simulink model "controllerSim"  (R2018b)
settings: Solver=VariableStepAuto  StartTime=0.0  StopTime=10.0  RelTol=1e-3
PreLoadFcn:
  | initParams;
values from neighbouring files (symbols this model uses):
  b = 3.508E-5    (= 3.508e-05)    [initParams.m]
  J = 3.228E-6    (= 3.228e-06)    [initParams.m]
  K = 2.740E-4    (= 0.000274)    [initParams.m]
  L = 2.750E-5    (= 2.75e-05)    [initParams.m]
  R = 4    [initParams.m]
undefined symbols (not defined in the file or in its folder): sigbuilder_block
libraries: simulink_extras x1
settings Model: Creator=cdsouza  LastModifiedBy=cdsouza
settings DebuggingCC: LibraryContextMissingDiagnostic=none
settings SFSimCC: SimUseLocalCustomCode=off
settings RTWCC: RTWUseLocalCustomCode=off

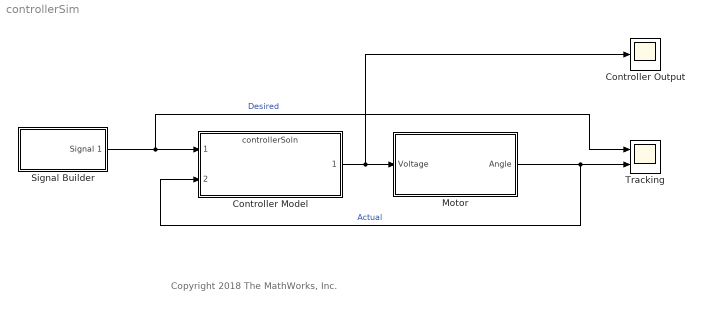
== system controllerSim ==
  note: Copyright 2018 The MathWorks, Inc.
  Controller Model : ModelReference  ModelNameDialog=controllerSoln  SimulationMode=Normal  ModelReferenceVersion=1.11
  Controller Output : Scope
  Motor : Subsystem  TreatAsAtomicUnit=on
  Signal Builder : Subsystem  Tag=STV Subsys  LoadFcn=sigbuilder_block('load');  StartFcn=sigbuilder_block('start');  StopFcn=sigbuilder_block('stop');  ClipboardFcn=sigbuilder_block('clipboard');  mask(Sigbuilder block){tuvar=[0:10]}
      mask help: Simulink:masks:SigbuilderBlock_MD
      mask init:
      | if ~strcmp(get_param(bdroot(gcbh),'SimulationStatus'),'stopped') tuvar = sigbuilder_block('maskInit'); end
      settings: CopyFcn=sigbuilder_block('copy');  DeleteFcn=sigbuilder_block('delete');  ModelCloseFcn=sigbuilder_block('modelClose');  PreSaveFcn=sigbuilder_block('preSave');  PauseFcn=sigbuilder_block('pause');  ContinueFcn=sigbuilder_block('continue');  NameChangeFcn=sigbuilder_block('namechange');  OpenFcn=sigbuilder_block('open',[436.966 199.241 549.931 400.345 ]);  CloseFcn=sigbuilder_block('close');
      mask Display: plot(0, 0, 100, 100,[2, 2, 32, 32, 2], [68, 8, 8, 68, 68],[32, 2], [38, 38], [32, 19, 2],[53, 60, 44], [32, 17, 17, 2],[16, 16, 31, 31]);txt = getActiveGroup(gcbh);text(2, 100, txt,'verticalAlignment', 'top');
  Tracking : Scope  NumInputPorts=2
  wires:
  Signal Builder/1(Signal 1) -> Tracking/1, Controller Model/1  "Desired"
  Motor/1(Angle) -> Controller Model/2, Tracking/2  "Actual"
  Controller Model/1 -> Controller Output/1, Motor/1(Voltage)

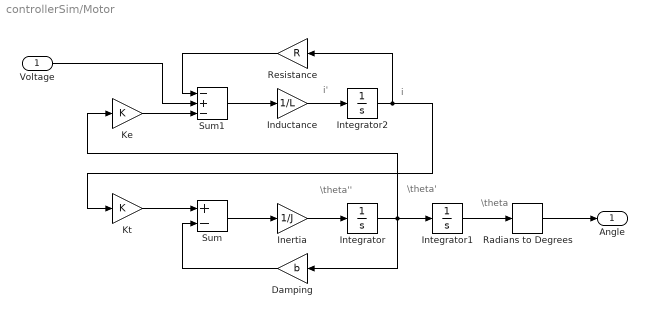
== system controllerSim/Motor ==
  note: \theta
  note: \theta''
  note: \theta'
  note: i
  note: i'
  Voltage : Inport
  Damping : Gain  Gain=b  SaturateOnIntegerOverflow=on  OutDataTypeStr=Inherit: Same as input  ParamDataTypeStr=Inherit: Same as input
  Inductance : Gain  Gain=1/L  SaturateOnIntegerOverflow=on  OutDataTypeStr=Inherit: Same as input  ParamDataTypeStr=Inherit: Same as input
  Inertia : Gain  Gain=1/J  SaturateOnIntegerOverflow=on  OutDataTypeStr=Inherit: Same as input  ParamDataTypeStr=Inherit: Same as input
  Integrator : Integrator
  Integrator1 : Integrator
  Integrator2 : Integrator
  Ke : Gain  Gain=K  SaturateOnIntegerOverflow=on  OutDataTypeStr=Inherit: Same as input  ParamDataTypeStr=Inherit: Same as input
  Kt : Gain  Gain=K  SaturateOnIntegerOverflow=on  OutDataTypeStr=Inherit: Same as input  ParamDataTypeStr=Inherit: Same as input
  Radians to Degrees : simulink_extras/Transformations/Radians to Degrees
  Resistance : Gain  Gain=R  SaturateOnIntegerOverflow=on  OutDataTypeStr=Inherit: Same as input  ParamDataTypeStr=Inherit: Same as input
  Sum : Sum  Inputs=+-  SaturateOnIntegerOverflow=on  InputSameDT=on  OutDataTypeStr=Inherit: Same as first input
  Sum1 : Sum  Inputs=-+-  SaturateOnIntegerOverflow=on  InputSameDT=on  OutDataTypeStr=Inherit: Same as first input
  Angle : Outport
  wires:
  Integrator/1 -> Damping/1, Integrator1/1, Ke/1
  Integrator2/1 -> Resistance/1, Kt/1
  Integrator1/1 -> Radians to Degrees/1
  Voltage/1 -> Sum1/2
  Resistance/1 -> Sum1/1
  Ke/1 -> Sum1/3
  Damping/1 -> Sum/2
  Kt/1 -> Sum/1
  Sum/1 -> Inertia/1
  Sum1/1 -> Inductance/1
  Inertia/1 -> Integrator/1
  Inductance/1 -> Integrator2/1
  Radians to Degrees/1 -> Angle/1

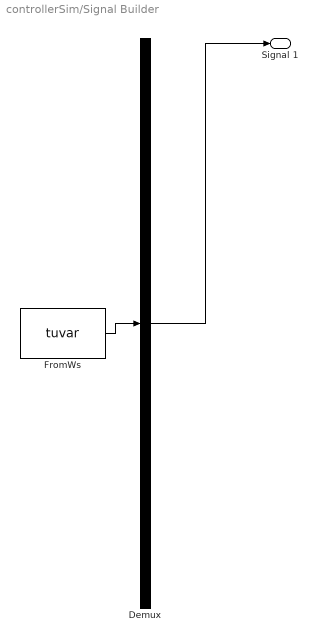
== system controllerSim/Signal Builder ==
  Demux : Demux  Tag=STV Demux  Outputs=1
  FromWs : FromWorkspace  Tag=STV FromWs  VariableName=tuvar  SampleTime=0
      SigBuilderData=|
      | common.afterFinalStr = 'Extrapolate'
      | common.sampleTime = 0
      | dataSet.timeRange = [0 25]
      | dataSet.name = 'Group 1'
      | sbobj.Groups.Name = 'Group 1'
      | sbobj.Groups.Signals.Name = 'Signal 1'
      | sbobj.Groups.Signals.XData = [0 1 4 6 10 15 20 25]
      | sbobj.Groups.Signals.YData = [0 60 30 80 40 30 20 -10]
      | sbobj.Groups.TimeRange = [0 25]
  Signal 1 : Outport  Tag=STV Outport
  wires:
  Demux/1 -> Signal 1/1
  FromWs/1 -> Demux/1
